simulink model "Simulation_5thJune"  (R2022b)
settings: Solver=VariableStepAuto  StartTime=0.0  StopTime=5  RelTol=1e-3
values from neighbouring files (symbols this model uses):
  C_f = 0.000112315*9    (= 0.001010835)    [Main.m]    (also in PSO_2paras.m = swarm(i,2); PSO_filter_2paras.m = swarm(i,2)/10000; Primary_test1.m; Script_18June.m = 0.0112315)
  f_c = 50e3    (= 50000)    [Main.m]    (also in Primary_test1.m; Script_18June.m; Script_23June.m; Script_5thJune.m)
  k = -0.5    [Main.m]    (also in Primary_test1.m; Savedata.m = 0.2909; Script_18June.m = 0.5; Script_23June.m)
  K_h11 = 0    [Main.m]    (also in PSO_HC.m = swarm(i,4); Primary_test1.m; Script_18June.m; Script_23June.m)
  K_h13 = 0    [Main.m]    (also in Primary_test1.m; Script_18June.m; Script_23June.m; Script_5thJune.m)
  K_h5 = 0    [Main.m]    (also in PSO_HC.m = swarm(i,1); Primary_test1.m = 1; Script_18June.m; Script_23June.m)
  K_h7 = 0    [Main.m]    (also in PSO_HC.m = swarm(i,2); Primary_test1.m; Script_18June.m; Script_23June.m)
  K_h9 = 0    [Main.m]    (also in PSO_HC.m = swarm(i,3); Script_18June.m; Script_23June.m; Script_5thJune.m)
  ki_pr = 160    [Main.m]    (also in PSO.m = swarm(i,2); Primary_test1.m; Savedata.m = 422.4716; Script_18June.m = 150)
  kL = 1e-7    (= 1e-07)    [Main.m]    (also in Primary_test1.m; Script_18June.m; Script_23June.m; Script_5thJune.m)
  Kp_pr = 1.7    [Main.m]    (also in PSO.m = swarm(i,1); Primary_test1.m; Savedata.m = 0.9028; Script_18June.m = 1)
  L_f = 0.000659829*1.4    (= 0.0009237606)    [Main.m]    (also in PSO_2paras.m = swarm(i,1); PSO_filter_2paras.m = swarm(i,1); Primary_test1.m; Script_18June.m = 0.000295603392)
  L_in1 = 0.35e-3    (= 0.00035)    [Main.m]    (also in Primary_test1.m; Script_18June.m; Script_23June.m; Script_5thJune.m)
  L_in2 = 0.35e-3    (= 0.00035)    [Main.m]    (also in Primary_test1.m; Script_18June.m; Script_23June.m; Script_5thJune.m)
  L_in3 = 0.35e-3    (= 0.00035)    [Main.m]    (also in Primary_test1.m; Script_18June.m; Script_23June.m; Script_5thJune.m)
  L_in4 = 0.35e-3    (= 0.00035)    [Main.m]    (also in Primary_test1.m; Script_18June.m; Script_23June.m; Script_5thJune.m)
  LD_ref1 = 100e-6    (= 0.0001)    [Main.m]    (also in Primary_test1.m; Script_18June.m = 5e-05; Script_23June.m = 1e-05; Script_5thJune.m = 1e-05)
  lo_co = 0.1    [Main.m]    (also in Primary_test1.m; Script_18June.m; Script_23June.m; Script_5thJune.m)
  m_p1 = 9.4e-5/droopDivide    (= 9.4e-06)    [Main.m]    (also in Primary_test1.m; Script_18June.m = 9.4e-05; Script_23June.m = 9.4e-05; Script_5thJune.m = 5e-05)
  m_p2 = 9.4e-5/droopDivide    (= 9.4e-06)    [Main.m]    (also in Primary_test1.m; Script_18June.m = 9.4e-05; Script_23June.m = 9.4e-05; Script_5thJune.m = 5e-05)
  m_p3 = 11.4e-5/droopDivide    (= 1.14e-05)    [Main.m]    (also in Primary_test1.m; Script_18June.m = 0.000114; Script_23June.m = 0.000114; Script_5thJune.m = 6.42857142857e-05)
  m_p4 = 11.4e-5/droopDivide    (= 1.14e-05)    [Main.m]    (also in Primary_test1.m; Script_18June.m = 0.000114; Script_23June.m = 0.000114; Script_5thJune.m = 6.42857142857e-05)
  n_q2 = 1.3e-3/droopDivide2    (= 6.5e-05)    [Main.m]    (also in Primary_test1.m; Script_18June.m; Script_23June.m; Script_5thJune.m = 0.2)
  n_q3 = 1.5e-3/droopDivide2    (= 7.5e-05)    [Main.m]    (also in Primary_test1.m; Script_18June.m; Script_23June.m; Script_5thJune.m = 0.257142857143)
  n_q4 = 1.5e-3/droopDivide2    (= 7.5e-05)    [Main.m]    (also in Primary_test1.m; Script_18June.m; Script_23June.m; Script_5thJune.m = 0.257142857143)
  R_f = 0.35    [Main.m]    (also in PSO_filter_2paras.m = 10*L_f; Primary_test1.m; Savedata.m = 0.249593207053; Script_18June.m = 0.1)
  R_in1 = 0.03    [Main.m]    (also in Primary_test1.m; Script_18June.m; Script_23June.m; Script_5thJune.m)
  R_in2 = 0.03    [Main.m]    (also in Primary_test1.m; Script_18June.m; Script_23June.m; Script_5thJune.m)
  R_in3 = 0.03    [Main.m]    (also in Primary_test1.m; Script_18June.m; Script_23June.m; Script_5thJune.m)
  R_in4 = 0.03    [Main.m]    (also in Primary_test1.m; Script_18June.m; Script_23June.m; Script_5thJune.m)
  Ts = 10e-6    (= 1e-05)    [Main.m]    (also in Primary_test1.m; Script_18June.m; Script_23June.m; Script_5thJune.m)
  V_nom = 220*sqrt(2)    [Main.m]    (also in Primary_test1.m; Script_18June.m; Script_23June.m; Script_5thJune.m)
  Vdc = 600    [Main.m]    (also in Primary_test1.m; Script_18June.m; Script_23June.m; Script_5thJune.m)
  w_c_high = 2*pi*50    (= 314.159265359)    [Main.m]    (also in Primary_test1.m; Script_18June.m = 307.876080052; Script_23June.m; Script_5thJune.m = 307.876080052)
  w_nom = 2*pi*f    (= 314.159265359)    [Main.m]    (also in Primary_test1.m; Script_18June.m; Script_23June.m; Script_5thJune.m)
  wc_hc = 1    [Main.m]    (also in Primary_test1.m; Script_18June.m = 0.3; Script_23June.m; Script_5thJune.m = 0.3)
  wc_pr = 3    [Main.m]    (also in PSO.m = swarm(i,3); Primary_test1.m; Savedata.m = 1.36672; Script_18June.m = 1.5)
undefined symbols (not defined in the file or in its folder): i
libraries: eeGeneralControl x16, spsThreePhaseSeriesRLCBranchLib x15, spsabctodq0Lib x14, spsabctoAlphaBetaZeroLib x13, spsThreePhaseVIMeasurementLib x12, slpidlib x8, spsDCVoltageSourceLib x4, spsAlphaBetaZerotoabcLib x4, spsSeriesRLCBranchLib x4, spsTriangleGeneratorLib x4, spsTwoLevelConverterLib x4, spsThreePhaseSeriesRLCLoadLib x2
(part 4 of 4)

== system Simulation_5thJune/Voltage Source Inverter 1/PLL_1p1/TienXuly ==
  v : Inport
  Gain : Gain  Gain=k
  Integrator : Integrator
  Integrator1 : Integrator
  Locthongthap : TransferFcn  Denominator=[1/fc2 1]
  Mux : Mux  Inputs=2
  Product : Product  RndMeth=Zero
  Product1 : Product  RndMeth=Zero
  Sum : Sum  Inputs=|+-
  Sum1 : Sum  Inputs=|+-
  Sum2 : Sum  Inputs=|+-
  v'-qv' : Scope
  wloc : Constant  Value=fc1*2*pi
  v' : Outport  VectorParamsAs1DForOutWhenUnconnected=off
  v'q : Outport  Port=2  VectorParamsAs1DForOutWhenUnconnected=off
  wires:
  Sum/1 -> Gain/1
  Gain/1 -> Sum1/1, Locthongthap/1
  Sum1/1 -> Product/1
  wloc/1 -> Product/2, Product1/1
  Product/1 -> Integrator/1
  Product1/1 -> Integrator1/1
  Integrator1/1 -> Sum1/2, Sum2/1
  Integrator/1 -> Product1/2, Sum/2, Mux/2, v'/1
  Locthongthap/1 -> Sum2/2
  v/1 -> Sum/1
  Sum2/1 -> v'q/1, Mux/1
  Mux/1 -> v'-qv'/1

== system Simulation_5thJune/Voltage Source Inverter 1/PLL_1p1/apha-beta=>dq ==
  Theta : Inport
  Uapha : Inport  Port=2
  Ubeta : Inport  Port=3
  Mux : Mux  Inputs=3
  Tinhvd : Fcn  Expr=(u[2]*cos(u[1])+u[3]*sin(u[1]))
  Tinhvq : Fcn  Expr=(-u[2]*sin(u[1])+u[3]*cos(u[1]))
  vq : Outport  VectorParamsAs1DForOutWhenUnconnected=off
  vd : Outport  Port=2  VectorParamsAs1DForOutWhenUnconnected=off
  wires:
  Theta/1 -> Mux/1
  Uapha/1 -> Mux/2
  Ubeta/1 -> Mux/3
  Mux/1 -> Tinhvd/1, Tinhvq/1
  Tinhvd/1 -> vd/1
  Tinhvq/1 -> vq/1

== system Simulation_5thJune/Voltage Source Inverter 1/PLL_1p2/TienXuly ==
  v : Inport
  Gain : Gain  Gain=k
  Integrator : Integrator
  Integrator1 : Integrator
  Locthongthap : TransferFcn  Denominator=[1/fc2 1]
  Mux : Mux  Inputs=2
  Product : Product  RndMeth=Zero
  Product1 : Product  RndMeth=Zero
  Sum : Sum  Inputs=|+-
  Sum1 : Sum  Inputs=|+-
  Sum2 : Sum  Inputs=|+-
  v'-qv' : Scope
  wloc : Constant  Value=fc1*2*pi
  v' : Outport  VectorParamsAs1DForOutWhenUnconnected=off
  v'q : Outport  Port=2  VectorParamsAs1DForOutWhenUnconnected=off
  wires:
  Sum/1 -> Gain/1
  Gain/1 -> Sum1/1, Locthongthap/1
  Sum1/1 -> Product/1
  wloc/1 -> Product/2, Product1/1
  Product/1 -> Integrator/1
  Product1/1 -> Integrator1/1
  Integrator1/1 -> Sum1/2, Sum2/1
  Integrator/1 -> Product1/2, Sum/2, Mux/2, v'/1
  Locthongthap/1 -> Sum2/2
  v/1 -> Sum/1
  Sum2/1 -> v'q/1, Mux/1
  Mux/1 -> v'-qv'/1

== system Simulation_5thJune/Voltage Source Inverter 1/PLL_1p2/apha-beta=>dq ==
  Theta : Inport
  Uapha : Inport  Port=2
  Ubeta : Inport  Port=3
  Mux : Mux  Inputs=3
  Tinhvd : Fcn  Expr=(u[2]*cos(u[1])+u[3]*sin(u[1]))
  Tinhvq : Fcn  Expr=(-u[2]*sin(u[1])+u[3]*cos(u[1]))
  vq : Outport  VectorParamsAs1DForOutWhenUnconnected=off
  vd : Outport  Port=2  VectorParamsAs1DForOutWhenUnconnected=off
  wires:
  Theta/1 -> Mux/1
  Uapha/1 -> Mux/2
  Ubeta/1 -> Mux/3
  Mux/1 -> Tinhvd/1, Tinhvq/1
  Tinhvd/1 -> vd/1
  Tinhvq/1 -> vq/1

== system Simulation_5thJune/Voltage Source Inverter 1/dq converter/Subsystem ==
  abc : Inport
  wt : Inport  Port=2
  Demux : Demux  Outputs=3
  abc to dq0 : spsabctodq0Lib/abc to dq0  Alignment=90 degrees behind phase A axis
  Out1 : Outport
  Out2 : Outport  Port=2
  wires:
  Demux/1 -> Out1/1
  abc to dq0/1 -> Demux/1
  wt/1 -> abc to dq0/2
  Demux/2 -> Out2/1
  abc/1 -> abc to dq0/1

== system Simulation_5thJune/Voltage Source Inverter 1/dq converter/Subsystem1 ==
  abc : Inport
  wt : Inport  Port=2
  Demux : Demux  Outputs=3
  abc to dq0 : spsabctodq0Lib/abc to dq0  Alignment=90 degrees behind phase A axis
  Out1 : Outport
  Out2 : Outport  Port=2
  wires:
  Demux/1 -> Out1/1
  abc to dq0/1 -> Demux/1
  wt/1 -> abc to dq0/2
  Demux/2 -> Out2/1
  abc/1 -> abc to dq0/1

== system Simulation_5thJune/Voltage Source Inverter 1/dq converter/Subsystem2 ==
  abc : Inport
  wt : Inport  Port=2
  Demux : Demux  Outputs=3
  abc to dq0 : spsabctodq0Lib/abc to dq0  Alignment=90 degrees behind phase A axis
  Out1 : Outport
  Out2 : Outport  Port=2
  wires:
  Demux/1 -> Out1/1
  abc to dq0/1 -> Demux/1
  wt/1 -> abc to dq0/2
  Demux/2 -> Out2/1
  abc/1 -> abc to dq0/1

== system Simulation_5thJune/Voltage Source Inverter 2/PLL_1p1/TienXuly ==
  v : Inport
  Gain : Gain  Gain=k
  Integrator : Integrator
  Integrator1 : Integrator
  Locthongthap : TransferFcn  Denominator=[1/fc2 1]
  Mux : Mux  Inputs=2
  Product : Product  RndMeth=Zero
  Product1 : Product  RndMeth=Zero
  Sum : Sum  Inputs=|+-
  Sum1 : Sum  Inputs=|+-
  Sum2 : Sum  Inputs=|+-
  v'-qv' : Scope
  wloc : Constant  Value=fc1*2*pi
  v' : Outport  VectorParamsAs1DForOutWhenUnconnected=off
  v'q : Outport  Port=2  VectorParamsAs1DForOutWhenUnconnected=off
  wires:
  Sum/1 -> Gain/1
  Gain/1 -> Sum1/1, Locthongthap/1
  Sum1/1 -> Product/1
  wloc/1 -> Product/2, Product1/1
  Product/1 -> Integrator/1
  Product1/1 -> Integrator1/1
  Integrator1/1 -> Sum1/2, Sum2/1
  Integrator/1 -> Product1/2, Sum/2, Mux/2, v'/1
  Locthongthap/1 -> Sum2/2
  v/1 -> Sum/1
  Sum2/1 -> v'q/1, Mux/1
  Mux/1 -> v'-qv'/1

== system Simulation_5thJune/Voltage Source Inverter 2/PLL_1p1/apha-beta=>dq ==
  Theta : Inport
  Uapha : Inport  Port=2
  Ubeta : Inport  Port=3
  Mux : Mux  Inputs=3
  Tinhvd : Fcn  Expr=(u[2]*cos(u[1])+u[3]*sin(u[1]))
  Tinhvq : Fcn  Expr=(-u[2]*sin(u[1])+u[3]*cos(u[1]))
  vq : Outport  VectorParamsAs1DForOutWhenUnconnected=off
  vd : Outport  Port=2  VectorParamsAs1DForOutWhenUnconnected=off
  wires:
  Theta/1 -> Mux/1
  Uapha/1 -> Mux/2
  Ubeta/1 -> Mux/3
  Mux/1 -> Tinhvd/1, Tinhvq/1
  Tinhvd/1 -> vd/1
  Tinhvq/1 -> vq/1

== system Simulation_5thJune/Voltage Source Inverter 2/PLL_1p2/TienXuly ==
  v : Inport
  Gain : Gain  Gain=k
  Integrator : Integrator
  Integrator1 : Integrator
  Locthongthap : TransferFcn  Denominator=[1/fc2 1]
  Mux : Mux  Inputs=2
  Product : Product  RndMeth=Zero
  Product1 : Product  RndMeth=Zero
  Sum : Sum  Inputs=|+-
  Sum1 : Sum  Inputs=|+-
  Sum2 : Sum  Inputs=|+-
  v'-qv' : Scope
  wloc : Constant  Value=fc1*2*pi
  v' : Outport  VectorParamsAs1DForOutWhenUnconnected=off
  v'q : Outport  Port=2  VectorParamsAs1DForOutWhenUnconnected=off
  wires:
  Sum/1 -> Gain/1
  Gain/1 -> Sum1/1, Locthongthap/1
  Sum1/1 -> Product/1
  wloc/1 -> Product/2, Product1/1
  Product/1 -> Integrator/1
  Product1/1 -> Integrator1/1
  Integrator1/1 -> Sum1/2, Sum2/1
  Integrator/1 -> Product1/2, Sum/2, Mux/2, v'/1
  Locthongthap/1 -> Sum2/2
  v/1 -> Sum/1
  Sum2/1 -> v'q/1, Mux/1
  Mux/1 -> v'-qv'/1

== system Simulation_5thJune/Voltage Source Inverter 2/PLL_1p2/apha-beta=>dq ==
  Theta : Inport
  Uapha : Inport  Port=2
  Ubeta : Inport  Port=3
  Mux : Mux  Inputs=3
  Tinhvd : Fcn  Expr=(u[2]*cos(u[1])+u[3]*sin(u[1]))
  Tinhvq : Fcn  Expr=(-u[2]*sin(u[1])+u[3]*cos(u[1]))
  vq : Outport  VectorParamsAs1DForOutWhenUnconnected=off
  vd : Outport  Port=2  VectorParamsAs1DForOutWhenUnconnected=off
  wires:
  Theta/1 -> Mux/1
  Uapha/1 -> Mux/2
  Ubeta/1 -> Mux/3
  Mux/1 -> Tinhvd/1, Tinhvq/1
  Tinhvd/1 -> vd/1
  Tinhvq/1 -> vq/1

== system Simulation_5thJune/Voltage Source Inverter 2/dq converter/Subsystem ==
  abc : Inport
  wt : Inport  Port=2
  Demux : Demux  Outputs=3
  abc to dq0 : spsabctodq0Lib/abc to dq0  Alignment=90 degrees behind phase A axis
  Out1 : Outport
  Out2 : Outport  Port=2
  wires:
  Demux/1 -> Out1/1
  abc to dq0/1 -> Demux/1
  wt/1 -> abc to dq0/2
  Demux/2 -> Out2/1
  abc/1 -> abc to dq0/1

== system Simulation_5thJune/Voltage Source Inverter 2/dq converter/Subsystem1 ==
  abc : Inport
  wt : Inport  Port=2
  Demux : Demux  Outputs=3
  abc to dq0 : spsabctodq0Lib/abc to dq0  Alignment=90 degrees behind phase A axis
  Out1 : Outport
  Out2 : Outport  Port=2
  wires:
  Demux/1 -> Out1/1
  abc to dq0/1 -> Demux/1
  wt/1 -> abc to dq0/2
  Demux/2 -> Out2/1
  abc/1 -> abc to dq0/1

== system Simulation_5thJune/Voltage Source Inverter 2/dq converter/Subsystem2 ==
  abc : Inport
  wt : Inport  Port=2
  Demux : Demux  Outputs=3
  abc to dq0 : spsabctodq0Lib/abc to dq0  Alignment=90 degrees behind phase A axis
  Out1 : Outport
  Out2 : Outport  Port=2
  wires:
  Demux/1 -> Out1/1
  abc to dq0/1 -> Demux/1
  wt/1 -> abc to dq0/2
  Demux/2 -> Out2/1
  abc/1 -> abc to dq0/1

== system Simulation_5thJune/Voltage Source Inverter 3/PLL_1p1/TienXuly ==
  v : Inport
  Gain : Gain  Gain=k
  Integrator : Integrator
  Integrator1 : Integrator
  Locthongthap : TransferFcn  Denominator=[1/fc2 1]
  Mux : Mux  Inputs=2
  Product : Product  RndMeth=Zero
  Product1 : Product  RndMeth=Zero
  Sum : Sum  Inputs=|+-
  Sum1 : Sum  Inputs=|+-
  Sum2 : Sum  Inputs=|+-
  v'-qv' : Scope
  wloc : Constant  Value=fc1*2*pi
  v' : Outport  VectorParamsAs1DForOutWhenUnconnected=off
  v'q : Outport  Port=2  VectorParamsAs1DForOutWhenUnconnected=off
  wires:
  Sum/1 -> Gain/1
  Gain/1 -> Sum1/1, Locthongthap/1
  Sum1/1 -> Product/1
  wloc/1 -> Product/2, Product1/1
  Product/1 -> Integrator/1
  Product1/1 -> Integrator1/1
  Integrator1/1 -> Sum1/2, Sum2/1
  Integrator/1 -> Product1/2, Sum/2, Mux/2, v'/1
  Locthongthap/1 -> Sum2/2
  v/1 -> Sum/1
  Sum2/1 -> v'q/1, Mux/1
  Mux/1 -> v'-qv'/1

== system Simulation_5thJune/Voltage Source Inverter 3/PLL_1p1/apha-beta=>dq ==
  Theta : Inport
  Uapha : Inport  Port=2
  Ubeta : Inport  Port=3
  Mux : Mux  Inputs=3
  Tinhvd : Fcn  Expr=(u[2]*cos(u[1])+u[3]*sin(u[1]))
  Tinhvq : Fcn  Expr=(-u[2]*sin(u[1])+u[3]*cos(u[1]))
  vq : Outport  VectorParamsAs1DForOutWhenUnconnected=off
  vd : Outport  Port=2  VectorParamsAs1DForOutWhenUnconnected=off
  wires:
  Theta/1 -> Mux/1
  Uapha/1 -> Mux/2
  Ubeta/1 -> Mux/3
  Mux/1 -> Tinhvd/1, Tinhvq/1
  Tinhvd/1 -> vd/1
  Tinhvq/1 -> vq/1

== system Simulation_5thJune/Voltage Source Inverter 3/PLL_1p2/TienXuly ==
  v : Inport
  Gain : Gain  Gain=k
  Integrator : Integrator
  Integrator1 : Integrator
  Locthongthap : TransferFcn  Denominator=[1/fc2 1]
  Mux : Mux  Inputs=2
  Product : Product  RndMeth=Zero
  Product1 : Product  RndMeth=Zero
  Sum : Sum  Inputs=|+-
  Sum1 : Sum  Inputs=|+-
  Sum2 : Sum  Inputs=|+-
  v'-qv' : Scope
  wloc : Constant  Value=fc1*2*pi
  v' : Outport  VectorParamsAs1DForOutWhenUnconnected=off
  v'q : Outport  Port=2  VectorParamsAs1DForOutWhenUnconnected=off
  wires:
  Sum/1 -> Gain/1
  Gain/1 -> Sum1/1, Locthongthap/1
  Sum1/1 -> Product/1
  wloc/1 -> Product/2, Product1/1
  Product/1 -> Integrator/1
  Product1/1 -> Integrator1/1
  Integrator1/1 -> Sum1/2, Sum2/1
  Integrator/1 -> Product1/2, Sum/2, Mux/2, v'/1
  Locthongthap/1 -> Sum2/2
  v/1 -> Sum/1
  Sum2/1 -> v'q/1, Mux/1
  Mux/1 -> v'-qv'/1

== system Simulation_5thJune/Voltage Source Inverter 3/PLL_1p2/apha-beta=>dq ==
  Theta : Inport
  Uapha : Inport  Port=2
  Ubeta : Inport  Port=3
  Mux : Mux  Inputs=3
  Tinhvd : Fcn  Expr=(u[2]*cos(u[1])+u[3]*sin(u[1]))
  Tinhvq : Fcn  Expr=(-u[2]*sin(u[1])+u[3]*cos(u[1]))
  vq : Outport  VectorParamsAs1DForOutWhenUnconnected=off
  vd : Outport  Port=2  VectorParamsAs1DForOutWhenUnconnected=off
  wires:
  Theta/1 -> Mux/1
  Uapha/1 -> Mux/2
  Ubeta/1 -> Mux/3
  Mux/1 -> Tinhvd/1, Tinhvq/1
  Tinhvd/1 -> vd/1
  Tinhvq/1 -> vq/1

== system Simulation_5thJune/Voltage Source Inverter 3/dq converter/Subsystem ==
  abc : Inport
  wt : Inport  Port=2
  Demux : Demux  Outputs=3
  abc to dq0 : spsabctodq0Lib/abc to dq0  Alignment=90 degrees behind phase A axis
  Out1 : Outport
  Out2 : Outport  Port=2
  wires:
  Demux/1 -> Out1/1
  abc to dq0/1 -> Demux/1
  wt/1 -> abc to dq0/2
  Demux/2 -> Out2/1
  abc/1 -> abc to dq0/1

== system Simulation_5thJune/Voltage Source Inverter 3/dq converter/Subsystem1 ==
  abc : Inport
  wt : Inport  Port=2
  Demux : Demux  Outputs=3
  abc to dq0 : spsabctodq0Lib/abc to dq0  Alignment=90 degrees behind phase A axis
  Out1 : Outport
  Out2 : Outport  Port=2
  wires:
  Demux/1 -> Out1/1
  abc to dq0/1 -> Demux/1
  wt/1 -> abc to dq0/2
  Demux/2 -> Out2/1
  abc/1 -> abc to dq0/1

== system Simulation_5thJune/Voltage Source Inverter 3/dq converter/Subsystem2 ==
  abc : Inport
  wt : Inport  Port=2
  Demux : Demux  Outputs=3
  abc to dq0 : spsabctodq0Lib/abc to dq0  Alignment=90 degrees behind phase A axis
  Out1 : Outport
  Out2 : Outport  Port=2
  wires:
  Demux/1 -> Out1/1
  abc to dq0/1 -> Demux/1
  wt/1 -> abc to dq0/2
  Demux/2 -> Out2/1
  abc/1 -> abc to dq0/1

== system Simulation_5thJune/Voltage Source Inverter 4/PLL_1p1/TienXuly ==
  v : Inport
  Gain : Gain  Gain=k
  Integrator : Integrator
  Integrator1 : Integrator
  Locthongthap : TransferFcn  Denominator=[1/fc2 1]
  Mux : Mux  Inputs=2
  Product : Product  RndMeth=Zero
  Product1 : Product  RndMeth=Zero
  Sum : Sum  Inputs=|+-
  Sum1 : Sum  Inputs=|+-
  Sum2 : Sum  Inputs=|+-
  v'-qv' : Scope
  wloc : Constant  Value=fc1*2*pi
  v' : Outport  VectorParamsAs1DForOutWhenUnconnected=off
  v'q : Outport  Port=2  VectorParamsAs1DForOutWhenUnconnected=off
  wires:
  Sum/1 -> Gain/1
  Gain/1 -> Sum1/1, Locthongthap/1
  Sum1/1 -> Product/1
  wloc/1 -> Product/2, Product1/1
  Product/1 -> Integrator/1
  Product1/1 -> Integrator1/1
  Integrator1/1 -> Sum1/2, Sum2/1
  Integrator/1 -> Product1/2, Sum/2, Mux/2, v'/1
  Locthongthap/1 -> Sum2/2
  v/1 -> Sum/1
  Sum2/1 -> v'q/1, Mux/1
  Mux/1 -> v'-qv'/1

== system Simulation_5thJune/Voltage Source Inverter 4/PLL_1p1/apha-beta=>dq ==
  Theta : Inport
  Uapha : Inport  Port=2
  Ubeta : Inport  Port=3
  Mux : Mux  Inputs=3
  Tinhvd : Fcn  Expr=(u[2]*cos(u[1])+u[3]*sin(u[1]))
  Tinhvq : Fcn  Expr=(-u[2]*sin(u[1])+u[3]*cos(u[1]))
  vq : Outport  VectorParamsAs1DForOutWhenUnconnected=off
  vd : Outport  Port=2  VectorParamsAs1DForOutWhenUnconnected=off
  wires:
  Theta/1 -> Mux/1
  Uapha/1 -> Mux/2
  Ubeta/1 -> Mux/3
  Mux/1 -> Tinhvd/1, Tinhvq/1
  Tinhvd/1 -> vd/1
  Tinhvq/1 -> vq/1

== system Simulation_5thJune/Voltage Source Inverter 4/PLL_1p2/TienXuly ==
  v : Inport
  Gain : Gain  Gain=k
  Integrator : Integrator
  Integrator1 : Integrator
  Locthongthap : TransferFcn  Denominator=[1/fc2 1]
  Mux : Mux  Inputs=2
  Product : Product  RndMeth=Zero
  Product1 : Product  RndMeth=Zero
  Sum : Sum  Inputs=|+-
  Sum1 : Sum  Inputs=|+-
  Sum2 : Sum  Inputs=|+-
  v'-qv' : Scope
  wloc : Constant  Value=fc1*2*pi
  v' : Outport  VectorParamsAs1DForOutWhenUnconnected=off
  v'q : Outport  Port=2  VectorParamsAs1DForOutWhenUnconnected=off
  wires:
  Sum/1 -> Gain/1
  Gain/1 -> Sum1/1, Locthongthap/1
  Sum1/1 -> Product/1
  wloc/1 -> Product/2, Product1/1
  Product/1 -> Integrator/1
  Product1/1 -> Integrator1/1
  Integrator1/1 -> Sum1/2, Sum2/1
  Integrator/1 -> Product1/2, Sum/2, Mux/2, v'/1
  Locthongthap/1 -> Sum2/2
  v/1 -> Sum/1
  Sum2/1 -> v'q/1, Mux/1
  Mux/1 -> v'-qv'/1

== system Simulation_5thJune/Voltage Source Inverter 4/PLL_1p2/apha-beta=>dq ==
  Theta : Inport
  Uapha : Inport  Port=2
  Ubeta : Inport  Port=3
  Mux : Mux  Inputs=3
  Tinhvd : Fcn  Expr=(u[2]*cos(u[1])+u[3]*sin(u[1]))
  Tinhvq : Fcn  Expr=(-u[2]*sin(u[1])+u[3]*cos(u[1]))
  vq : Outport  VectorParamsAs1DForOutWhenUnconnected=off
  vd : Outport  Port=2  VectorParamsAs1DForOutWhenUnconnected=off
  wires:
  Theta/1 -> Mux/1
  Uapha/1 -> Mux/2
  Ubeta/1 -> Mux/3
  Mux/1 -> Tinhvd/1, Tinhvq/1
  Tinhvd/1 -> vd/1
  Tinhvq/1 -> vq/1

== system Simulation_5thJune/Voltage Source Inverter 4/dq converter/Subsystem ==
  abc : Inport
  wt : Inport  Port=2
  Demux : Demux  Outputs=3
  abc to dq0 : spsabctodq0Lib/abc to dq0  Alignment=90 degrees behind phase A axis
  Out1 : Outport
  Out2 : Outport  Port=2
  wires:
  Demux/1 -> Out1/1
  abc to dq0/1 -> Demux/1
  wt/1 -> abc to dq0/2
  Demux/2 -> Out2/1
  abc/1 -> abc to dq0/1

== system Simulation_5thJune/Voltage Source Inverter 4/dq converter/Subsystem1 ==
  abc : Inport
  wt : Inport  Port=2
  Demux : Demux  Outputs=3
  abc to dq0 : spsabctodq0Lib/abc to dq0  Alignment=90 degrees behind phase A axis
  Out1 : Outport
  Out2 : Outport  Port=2
  wires:
  Demux/1 -> Out1/1
  abc to dq0/1 -> Demux/1
  wt/1 -> abc to dq0/2
  Demux/2 -> Out2/1
  abc/1 -> abc to dq0/1

== system Simulation_5thJune/Voltage Source Inverter 4/dq converter/Subsystem2 ==
  abc : Inport
  wt : Inport  Port=2
  Demux : Demux  Outputs=3
  abc to dq0 : spsabctodq0Lib/abc to dq0  Alignment=90 degrees behind phase A axis
  Out1 : Outport
  Out2 : Outport  Port=2
  wires:
  Demux/1 -> Out1/1
  abc to dq0/1 -> Demux/1
  wt/1 -> abc to dq0/2
  Demux/2 -> Out2/1
  abc/1 -> abc to dq0/1
